simulink model "Crane_Model_Simulink"  (R2023a)
settings: Solver=FixedStepAuto  StartTime=0.0  StopTime=stop_time  FixedStep=1/1000  RelTol=1e-3
values from neighbouring files (symbols this model uses):
  F_max = P_max / V_max    (= 4500)    [Crane_Sway_Control.m]
  g = 9.81    [Crane_Sway_Control.m]
  K = lqr(A,B,Q,R)    [Crane_Sway_Control.m]
  l = 3    [Crane_Sway_Control.m]
  m = 5    [Crane_Sway_Control.m]
  M = 250    [Crane_Sway_Control.m]
libraries: slpidlib x1
settings Model: Creator=LENOVO THINKPAD  LastModifiedBy=LENOVO THINKPAD

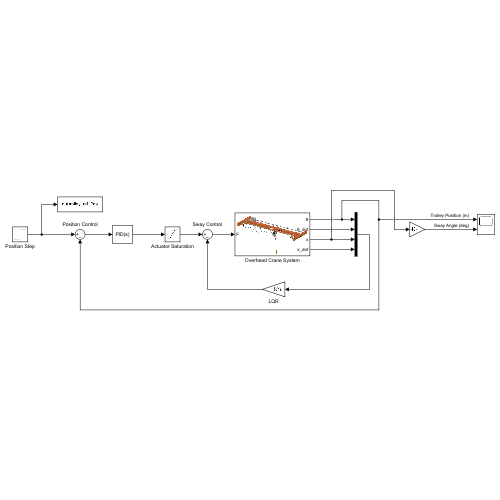
[thumbnail: Simulink's stored preview of the top-level diagram]
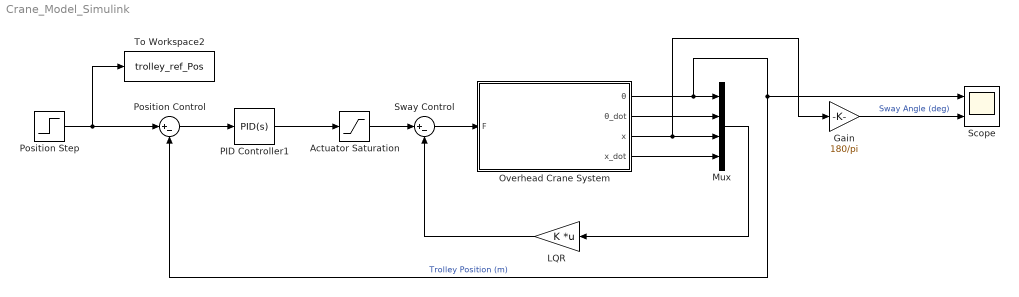
== system Crane_Model_Simulink ==
  Actuator Saturation : Saturate  UpperLimit=F_max  LowerLimit=-F_max
  Gain : Gain  Gain=180/pi
  LQR : Gain  Gain=K  Multiplication=Matrix(K*u)
  Mux : Mux
  Overhead Crane System : Subsystem
      mask Display: image('$imagefile'); % Use "Edit Image" on toolstrip to change.
  PID Controller1 : slpidlib/PID Controller  Controller=PID  Form=Parallel  TimeDomain=Continuous-time  UseExternalTs=off  SampleTime=-1  IntegratorMethod=Forward Euler  FilterMethod=Forward Euler  ControllerParametersSource=internal  P=50  I=0.15  UseKiTs=off  D=250  N=100  UseFilter=on  TunerSelectOption=Transfer Function Based (PID Tuner App)  InitialConditionSource=internal  InitialConditionForIntegrator=0  InitialConditionForFilter=0  DifferentiatorICPrevScaledInput=0  ExternalReset=none  TrackingMode=off  Kt=1  LimitOutput=off  SatLimitsSource=internal  UpperSaturationLimit=inf  LowerSaturationLimit=-inf  LinearizeAsGain=on  AntiWindupMode=none  Kb=1  LimitIntegrator=off  UpperIntegratorSaturationLimit=inf  LowerIntegratorSaturationLimit=-inf  POutMin=[]  POutMax=[]  IOutMin=[]  IOutMax=[]  DOutMin=[]  DOutMax=[]  NOutMin=[]  NOutMax=[]  SumOutMin=[]  SumOutMax=[]  SaturationOutMin=[]  SaturationOutMax=[]  PParamMin=[]  PParamMax=[]  IParamMin=[]  IParamMax=[]  DParamMin=[]  DParamMax=[]  NParamMin=[]  NParamMax=[]  KbParamMin=[]  KbParamMax=[]  KtParamMin=[]  KtParamMax=[]  KbOutMin=[]  KbOutMax=[]  KtOutMin=[]  KtOutMax=[]  IntegratorOutMin=[]  IntegratorOutMax=[]  FilterOutMin=[]  FilterOutMax=[]  SumI1OutMin=[]  SumI1OutMax=[]  SumI2OutMin=[]  SumI2OutMax=[]  SumI3OutMin=[]  SumI3OutMax=[]  SumI4OutMin=[]  SumI4OutMax=[]  SumDOutMin=[]  SumDOutMax=[]  DifferentiatorOutMin=[]  DifferentiatorOutMax=[]  FilterDiffOutCoefMin=[]  FilterDiffOutCoefMax=[]  ReciprocalOutMin=[]  ReciprocalOutMax=[]  SumDenOutMin=[]  SumDenOutMax=[]  SumNumOutMin=[]  SumNumOutMax=[]  DivideOutMin=[]  DivideOutMax=[]  UdiffTsProdOutMin=[]  UdiffTsProdOutMax=[]  NTsProdOutMin=[]  NTsProdOutMax=[]  UintegralTsProdOutMin=[]  UintegralTsProdOutMax=[]  UngainTsProdOutMin=[]  UngainTsProdOutMax=[]  ClampingZeroOutDataTypeStr=Inherit: Inherit via back propagation  ClampingZeroOutMin=[]  ClampingZeroOutMax=[]  FilterDenConstantOutDataTypeStr=Inherit: Inherit via back propagation  FilterDenConstantOutMin=[]  FilterDenConstantOutMax=[]  PCopyOutDataTypeStr=Inherit: Inherit via back propagation  PCopyOutMin=[]  PCopyOutMax=[]  NCopyOutDataTypeStr=Inherit: Inherit via back propagation  NCopyOutMin=[]  NCopyOutMax=[]  IntegratorContinuousStateAttributes=''  IntegratorStateMustResolveToSignalObject=off  IntegratorRTWStateStorageClass=Auto  FilterContinuousStateAttributes=''  FilterStateMustResolveToSignalObject=off  FilterRTWStateStorageClass=Auto  ParallelPVariant=InternalParameters  IdealPVariant=Disabled  IVariant=InternalParameters  DVariant=InternalParameters  IntegratorVariant=Continuous  SatVariant=Disabled  AWVariant=Passthrough  PCopyVariant=Disabled  TRVariant=Disabled  FdbkBlocksVariant=Forward  IdealPFdbkVariant=Disabled  SatFdbkVariant=Disabled  DerivativeFilterVariant=ContFilter  NVariant=InternalParameters  NCopyVariant=Disabled  FilterICVariant=InternalICsFilter  IntegratorICVariant=InternalICs  ExternalResetVariant=Disabled  TRSumVariant=Passthrough  SumFdbkVariant=Disabled  SumVariant=Sum_PID  TsampFilterVariant=InternalTs  TsampNgainVariant=Passthrough  TsampIntegralVariant=Disabled_SignalSpec  ExternalSaturationOutDataTypeStr=Inherit: Same as second input
  Position Control : Sum  Inputs=|+-
  Position Step : Step  Time=0  After=4  SampleTime=0
  Scope : Scope  NumInputPorts=2
  Sway Control : Sum  Inputs=|+-
  To Workspace2 : ToWorkspace  VariableName=trolley_ref_Pos  SaveFormat=Timeseries  SampleTime=-1
  wires:
  Position Control/1 -> PID Controller1/1
  PID Controller1/1 -> Actuator Saturation/1
  Position Step/1 -> Position Control/1, To Workspace2/1
  Actuator Saturation/1 -> Sway Control/1
  Sway Control/1 -> Overhead Crane System/1(F)
  Mux/1 -> LQR/1
  LQR/1 -> Sway Control/2
  Gain/1 -> Scope/2  "Sway Angle (deg)"
  Overhead Crane System/4(x_dot) -> Mux/4
  Overhead Crane System/3(x) -> Mux/3, Gain/1
  Overhead Crane System/2(θ_dot) -> Mux/2
  Overhead Crane System/1(θ) -> Position Control/2, Scope/1, Mux/1  "Trolley Position (m)"

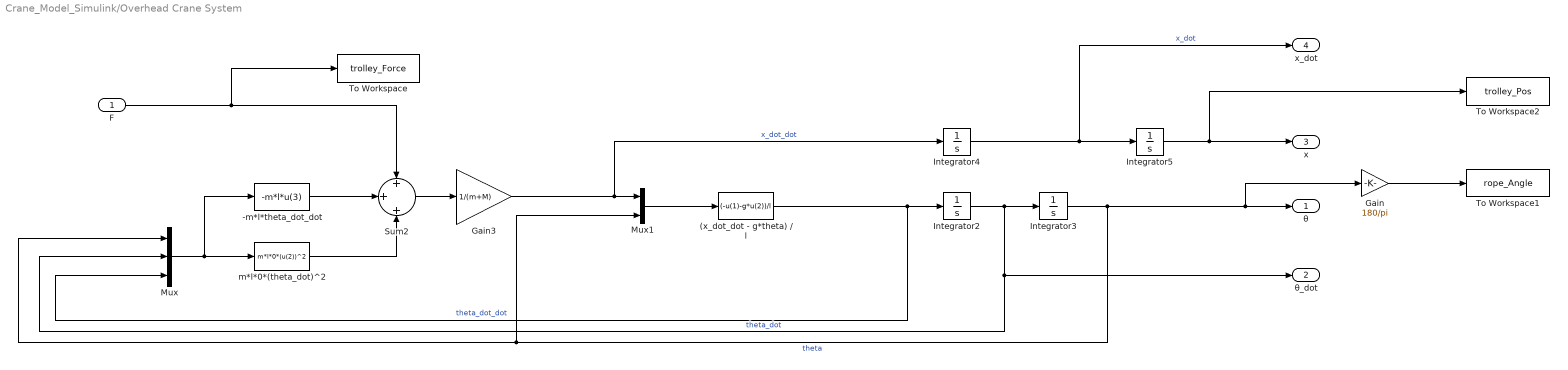
== system Crane_Model_Simulink/Overhead Crane System ==
  F : Inport
  (x_dot_dot - g*theta) / l : Fcn  Expr=(-u(1)-g*u(2))/l
  -m*l*theta_dot_dot : Fcn  Expr=-m*l*u(3)
  Gain : Gain  Gain=180/pi
  Gain3 : Gain  Gain=1/(m+M)
  Integrator{2..5} (4 alike) : Integrator
  Mux : Mux  Inputs=3
  Mux1 : Mux  Inputs=2
  Sum2 : Sum  Inputs=+|+|+
  To Workspace : ToWorkspace  VariableName=trolley_Force  SaveFormat=Timeseries  SampleTime=-1
  To Workspace1 : ToWorkspace  VariableName=rope_Angle  SaveFormat=Timeseries  SampleTime=-1
  To Workspace2 : ToWorkspace  VariableName=trolley_Pos  SaveFormat=Timeseries  SampleTime=-1
  m*l*0*(theta_dot)^2 : Fcn  Expr=m*l*0*(u(2))^2
  θ : Outport
  θ_dot : Outport  Port=2
  x : Outport  Port=3
  x_dot : Outport  Port=4
  wires:
  F/1 -> Sum2/1, To Workspace/1
  Gain/1 -> To Workspace1/1
  Gain3/1 -> Integrator4/1, Mux1/1  "x_dot_dot"
  Integrator4/1 -> Integrator5/1, x_dot/1  "x_dot"
  Integrator3/1 -> Gain/1, θ/1, Mux/1, Mux1/2  "theta"
  Sum2/1 -> Gain3/1
  (x_dot_dot - g*theta) / l/1 -> Mux/3, Integrator2/1  "theta_dot_dot"
  Integrator2/1 -> Mux/2, θ_dot/1, Integrator3/1  "theta_dot"
  -m*l*theta_dot_dot/1 -> Sum2/2
  Mux/1 -> -m*l*theta_dot_dot/1, m*l*0*(theta_dot)^2/1
  m*l*0*(theta_dot)^2/1 -> Sum2/3
  Mux1/1 -> (x_dot_dot - g*theta) / l/1
  Integrator5/1 -> To Workspace2/1, x/1
